simulink model "ExampleOpponentStates"  (Simulink 9.2)
settings: Solver=FixedStepDiscrete  StartTime=0.0  StopTime=inf  FixedStep=0.001  RelTol=1e-3  EnableMultiTasking=on
PostLoadFcn:
  | TIMESTEP = 0.001;
libraries: rFproPhysicsLib x6, simulink x1
settings Model: Creator=enewton  LastModifiedBy=SeanKavanagh
settings OptimizationCC: ExpressionDepthLimit=2147483647
settings DebuggingCC: SolverPrmCheckMsg=warning
settings RTWCC: SystemTargetFile=rfpro.tlc  MakeCommand="make_rtw OPTS=\"-DRUN_PHYSICS\""  TemplateMakefile=rfpro.tmf  Description=rFpro Target (Run Physics)  TargetLang=C++
settings STFCustomTargetCC: ModelReferenceCompliant=off  GeneratePreprocessorConditionals=Disable all  CombineOutputUpdateFcns=on  MatFileLogging=on  CPPClassGenCompliant=on  GRTInterface=off  SystemTargetFile=rfpro.tlc
settings GRTTargetCC: ModelReferenceCompliant=off  ParMdlRefBuildCompliant=off  CompOptLevelCompliant=off  ConcurrentExecutionCompliant=off  CombineOutputUpdateFcns=on  GRTInterface=off  UseToolchainInfoCompliant=off

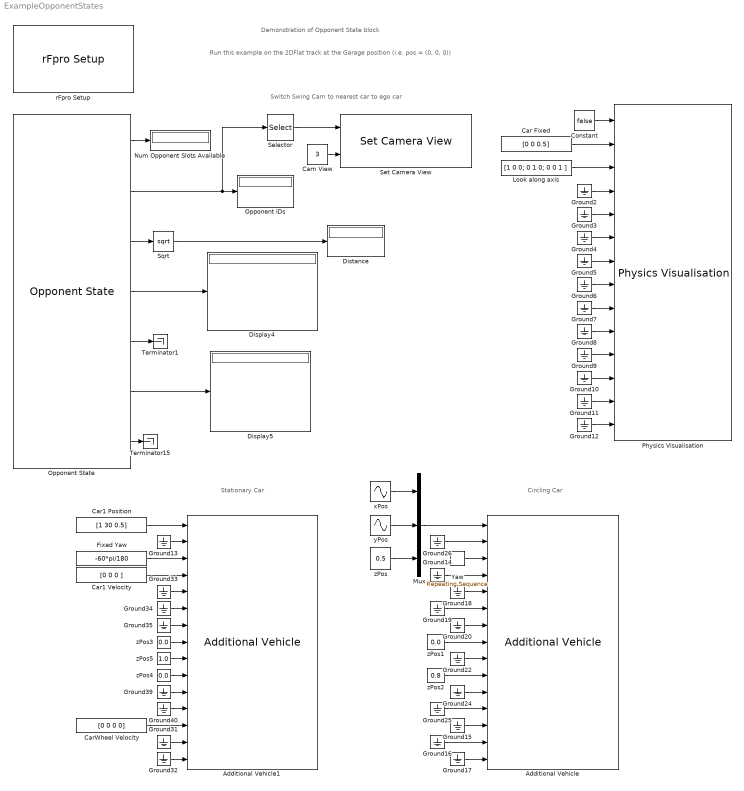
== system ExampleOpponentStates ==
  note: Run this example on the 2DFlat track at the Garage position (i.e. pos = (0, 0, 0))
  note: Switch Swing Cam to nearest car to ego car
  note: Circling Car
  note: Stationary Car
  note: Demonstration of Opponent State block
  Additional Vehicle : rFproPhysicsLib/Additional Vehicle  VEH_FILE='Hatchback_AWD_Blue'  DRIVER_NAME=''  UPGRADE_PACK=0  SKIN=''  HELMET=''  COLLIDABLE=off  TRANSPARENT_PROXIMITY=0  MANUAL_TRANSPARENCY=0  HEIGHT_VALID=on  ORI_VALID=off  HEADING_VALID=on  VEL_VALID=off  ROT_VALID=off  GEAR_VALID=off  RPM_VALID=off  INPUTS_VALID=on  BRAKE_LIGHT_VALID=off  HEADLIGHT_VALID=off  WHEEL_ROTATIONS_VALID=off  WHEEL_BRAKE_TEMPS_VALID=off  WHEEL_HEIGHTS_VALID=off  period=0.01  offset=0  useReverseByteOrder=on  rFpro__platform=Remote Model - Default
  Additional Vehicle1 : rFproPhysicsLib/Additional Vehicle  VEH_FILE='Hatchback_AWD_White'  DRIVER_NAME=''  UPGRADE_PACK=0  SKIN=''  HELMET=''  COLLIDABLE=off  TRANSPARENT_PROXIMITY=0  MANUAL_TRANSPARENCY=0  HEIGHT_VALID=on  ORI_VALID=off  HEADING_VALID=on  VEL_VALID=on  ROT_VALID=off  GEAR_VALID=off  RPM_VALID=off  INPUTS_VALID=on  BRAKE_LIGHT_VALID=off  HEADLIGHT_VALID=off  WHEEL_ROTATIONS_VALID=on  WHEEL_BRAKE_TEMPS_VALID=off  WHEEL_HEIGHTS_VALID=off  period=0.01  offset=0  useReverseByteOrder=on  rFpro__platform=Remote Model - Default
  Cam View : Constant  Value=3
  Car Fixed : Constant  Value=[0 0 0.5]
  Car1 Position : Constant  Value=[1 30 0.5]
  Car1 Velocity : Constant  Value=[0 0 0 ]
  CarWheel Velocity : Constant  Value=[0 0 0 0]
  Constant : Constant  Value=false
  Display4 : Display
  Display5 : Display
  Distance : Display
  Fixed Yaw : Constant  Value=-60*pi/180
  Ground{2..20,22,24..26,31..35,39..40} (30 alike) : Ground
  Look along axis : Constant  Value=[1 0 0; 0 1 0; 0 0 1 ]
  Mux : Mux  Inputs=3
  Num Opponent Slots Available : Display
  Opponent IDs : Display
  Opponent State : rFproPhysicsLib/Opponent State  max_SL_opponents=2  flattenOutput=on
  Physics Visualisation : rFproPhysicsLib/Physics Visualisation  PAR_SKIP_INTERNAL_PHYSICS=off  PAR_ACCEL_VALID=off  PAR_ROT_ACCEL_VALID=off  PAR_GEAR_VALID=off  PAR_RPM_VALID=off  PAR_INPUTS_VALID=off  PAR_STEER_TORQUE_VALID=off  PAR_HEADLIGHTS_ON_VALID=off  PAR_WHEEL_POS_VALID=off  PAR_WHEEL_ORI_VALID=off  PAR_TYRE_PARAMS_VALID=off  PAR_WHEEL_ROTATION_VALID=off  PAR_WHEEL_BRAKE_TEMP_VALID=off  PAR_WHEEL_TREAD_TEMP_VALID=off  PAR_WHEEL_AIR_TEMP_VALID=off  period=-1  offset=0  useReverseByteOrder=on  rFpro__platform=Remote Model - Default
  Selector : Selector  InputPortWidth=2  IndexOptions=Index vector (dialog)  Indices=[1]  OutputSizes=1
  Set Camera View : rFproPhysicsLib/Set Camera View  triggerWidth=1  useReverseByteOrder=off  rFpro__platform=Remote Model - Default
  Sqrt : Sqrt  SaturateOnIntegerOverflow=on
  Terminator1 : Terminator
  Terminator15 : Terminator
  Yaw : simulink/Sources/Repeating Sequence  rep_seq_t=[0 6]  rep_seq_y=[0 -2*pi]
  rFpro Setup : rFproPhysicsLib/rFpro Setup  platform=Remote Model - Default  stopOnSessionEnd=on  usePseudoRealtime=on  syncToRF=on  useReverseByteOrder=off  useRfTime=on  minIterations=4  maxIterations=1000  ipReceiveAddress='127.0.0.1'  ipReceivePort=11054  receiveSampleTime=-1  ipTransmitAddress='127.0.0.1'  ipTransmitPort=11052  transmitSampleTime=-1  pluginType=RUN_PHYSICS  sysTarget=xpctarget.tlc  templateMakeFile=xpc_default_tmf  makeCommand=make_rtw  buildDesc=xPC target
  xPos : Sin  Amplitude=20  Bias=30  Frequency=2*pi/6  SampleTime=0
  yPos : Sin  Amplitude=20  Frequency=2*pi/6  Phase=pi/2  SampleTime=0
  zPos : Constant  Value=0.5
  zPos1 : Constant  Value=0.0
  zPos2 : Constant  Value=0.8
  zPos3 : Constant  Value=0.0
  zPos4 : Constant  Value=0.0
  zPos5 : Constant  Value=1.0
  wires:
  Constant/1 -> Physics Visualisation/1
  Car Fixed/1 -> Physics Visualisation/2
  Look along axis/1 -> Physics Visualisation/3
  Ground2/1 -> Physics Visualisation/4
  Ground3/1 -> Physics Visualisation/5
  Ground4/1 -> Physics Visualisation/6
  Ground5/1 -> Physics Visualisation/7
  Ground6/1 -> Physics Visualisation/8
  Ground7/1 -> Physics Visualisation/9
  Ground8/1 -> Physics Visualisation/10
  Ground9/1 -> Physics Visualisation/11
  Ground10/1 -> Physics Visualisation/12
  Ground11/1 -> Physics Visualisation/13
  Opponent State/2 -> Selector/1, Opponent IDs/1
  Sqrt/1 -> Distance/1
  Ground12/1 -> Physics Visualisation/14
  Ground17/1 -> Additional Vehicle/15
  Ground16/1 -> Additional Vehicle/14
  Ground15/1 -> Additional Vehicle/13
  Ground25/1 -> Additional Vehicle/12
  Ground24/1 -> Additional Vehicle/11
  zPos2/1 -> Additional Vehicle/10
  Ground22/1 -> Additional Vehicle/9
  zPos1/1 -> Additional Vehicle/8
  Ground20/1 -> Additional Vehicle/7
  Ground19/1 -> Additional Vehicle/6
  Ground18/1 -> Additional Vehicle/5
  Ground14/1 -> Additional Vehicle/4
  Yaw/1 -> Additional Vehicle/3
  Mux/1 -> Additional Vehicle/1
  Opponent State/3 -> Sqrt/1
  Ground32/1 -> Additional Vehicle1/15
  Ground31/1 -> Additional Vehicle1/14
  CarWheel Velocity/1 -> Additional Vehicle1/13
  Ground40/1 -> Additional Vehicle1/12
  Ground39/1 -> Additional Vehicle1/11
  zPos4/1 -> Additional Vehicle1/10
  zPos5/1 -> Additional Vehicle1/9
  zPos3/1 -> Additional Vehicle1/8
  Ground35/1 -> Additional Vehicle1/7
  Ground34/1 -> Additional Vehicle1/6
  Ground33/1 -> Additional Vehicle1/5
  Car1 Velocity/1 -> Additional Vehicle1/4
  Fixed Yaw/1 -> Additional Vehicle1/3
  Car1 Position/1 -> Additional Vehicle1/1
  xPos/1 -> Mux/1
  yPos/1 -> Mux/2
  zPos/1 -> Mux/3
  Ground26/1 -> Additional Vehicle/2
  Opponent State/1 -> Num Opponent Slots Available/1
  Opponent State/5 -> Terminator1/1
  Opponent State/6 -> Display5/1
  Opponent State/7 -> Terminator15/1
  Cam View/1 -> Set Camera View/2
  Selector/1 -> Set Camera View/1
  Opponent State/4 -> Display4/1
  Ground13/1 -> Additional Vehicle1/2
